simulink model "power_triphaseline"  (Simulink 6.0)
settings: Solver=ode15s  SolverMode=SingleTasking  StartTime=0.0  StopTime=0.1  RelTol=1e-3  AbsTol=1e-6
libraries: powerlib x17
settings Model: Creator=patrice  LastModifiedBy=batserve  ExtModeTrigMode=oneshot  ExtModeArmWhenConnect=off  ExtModeAutoUpdateStatusClock=off
settings DataIOCC: LimitDataPoints=off  SignalLoggingName=sigsOut
settings OptimizationCC: BlockReduction=off  BooleanDataType=off
settings DebuggingCC: CheckExecutionContextPreStartOutputMsg=on  CheckExecutionContextRuntimeOutputMsg=on  SolverPrmCheckMsg=none  IntegerOverflowMsg=none
settings HardwareCC: TargetUnknown=on
settings RTWCC: TemplateMakefile=grt_unix.tmf

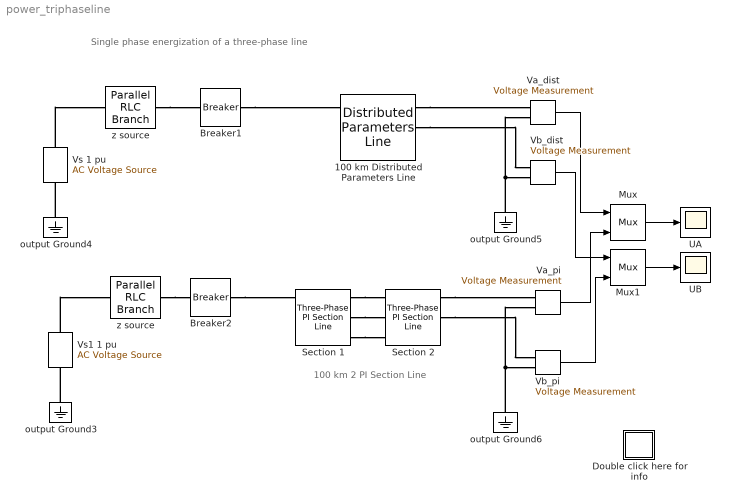
== system power_triphaseline ==
  note: 100 km
      | 2 PI Section Line
  note: Single phase energization of a three-phase line
  100 km Distributed Parameters Line : powerlib/Elements/Distributed Parameters Line  Phases=3  Frequency=60  Resistance=[0.01273 0.3864]  Inductance="[0.9337e-3  4.1264e-3]"  Capacitance=[12.74e-9 7.751e-9]  Length=100  x1=[0 0 0 0; 0.0001244 0 0 0; 0.0002488 0 0 0; 0.0003733 0 0 0; 0.0004977 0 0 0; 0.0006221 0 0 0]  x2=[0 0 0 0; 0.0001244 0 0 0; 0.0002488 0 0 0; 0.0003733 0 0 0; 0.0004977 0 0 0; 0.0006221 0 0 0]  x3=[0 0 0 0; 0.0001244 0 0 0; 0.0002488 0 0 0; 0.0003733 0 0 0; 0.0004977 0 0 0; 0.0006221 0 0 0]  x4=[0 0 0 0; 0.0001244 0 0 0; 0.0002488 0 0 0; 0.0003733 0 0 0; 0.0004977 0 0 0; 0.0006221 0 0 0]  x5=0  Measurements=None
      settings: AttributesFormatString=\n
  Breaker1 : powerlib/Elements/Breaker  BreakerResistance=0.01  InitialState=0  SnubberResistance=inf  SnubberCapacitance=0  SwitchingTimes="[ 0.25/60  4/60 ]"  External=off  Measurements=None
      settings: AttributesFormatString=\n
  Breaker2 : powerlib/Elements/Breaker  BreakerResistance=0.01  InitialState=0  SnubberResistance=inf  SnubberCapacitance=0  SwitchingTimes="[ .25/60  4/60 ]"  External=off  Measurements=None
      settings: AttributesFormatString=\n
  Double click here for info : Subsystem
      mask Display: disp('?')
  Mux : Mux  Inputs=2
  Mux1 : Mux  Inputs=2
  Section 1 : powerlib/Elements/Three-Phase PI Section Line  PhysicalDomain=powersysdomain  SubClassName=unknown  LeftPortType=p1  RightPortType=p1  LConnTagsString=a|b|c  RConnTagsString=A|B|C  Frequency=60  Resistances=[ 0.01273 0.3864]  Inductances="[ 0.9337e-3  4.1264e-3]"  Capacitances=[12.74e-9 7.751e-9]  Length=50
  Section 2 : powerlib/Elements/Three-Phase PI Section Line  PhysicalDomain=powersysdomain  SubClassName=unknown  LeftPortType=p1  RightPortType=p1  LConnTagsString=a|b|c  RConnTagsString=A|B|C  Frequency=60  Resistances=[ 0.01273 0.3864]  Inductances="[ 0.9337e-3  4.1264e-3]"  Capacitances=[12.74e-9 7.751e-9]  Length=50
  UA : Scope
      settings: TickLabels=on  TimeRange=0.1  YMin=-4  YMax=4  DataFormat=Array
  UB : Scope
      settings: TickLabels=on  TimeRange=0.1  YMin=-1  YMax=1  DataFormat=Array  MaxDataPoints=500000
  Va_dist : powerlib/Measurements/Voltage Measurement  Tag=PoWeRsYsTeMmEaSuReMeNt  PhasorSimulation=off  OutputType=Magnitude  PSBequivalent=0
  Va_pi : powerlib/Measurements/Voltage Measurement  Tag=PoWeRsYsTeMmEaSuReMeNt  PhasorSimulation=off  OutputType=Magnitude  PSBequivalent=0
  Vb_dist : powerlib/Measurements/Voltage Measurement  Tag=PoWeRsYsTeMmEaSuReMeNt  PhasorSimulation=off  OutputType=Magnitude  PSBequivalent=0
  Vb_pi : powerlib/Measurements/Voltage Measurement  Tag=PoWeRsYsTeMmEaSuReMeNt  PhasorSimulation=off  OutputType=Magnitude  PSBequivalent=0
  Vs 1 pu : powerlib/Electrical Sources/AC Voltage Source  Description=source block  Orientation=up  Amplitude=1  Phase=0  Frequency=60  SampleTime=0  Measurements=None
      settings: AttributesFormatString=\n
  Vs1 1 pu : powerlib/Electrical Sources/AC Voltage Source  Description=source block  Orientation=up  Amplitude=1  Phase=0  Frequency=60  SampleTime=0  Measurements=None
      settings: AttributesFormatString=\n
  output Ground{3..6} (4 alike) : powerlib/Elements/Ground  Orientation=down  PhysicalDomain=powersysdomain  SubClassName=unknown  LeftPortType=p1  RightPortType=p1  LConnTagsString=a
  z source : powerlib/Elements/Parallel RLC Branch  PhysicalDomain=powersysdomain  SubClassName=unknown  LeftPortType=p1  RightPortType=p1  LConnTagsString=a  RConnTagsString=__new0  Resistance=180  Inductance=47.8e-3  Capacitance=0  Measurements=None
  "z source " : powerlib/Elements/Parallel RLC Branch  PhysicalDomain=powersysdomain  SubClassName=unknown  LeftPortType=p1  RightPortType=p1  LConnTagsString=a  RConnTagsString=__new0  Resistance=180  Inductance=47.8e-3  Capacitance=0  Measurements=None
  wires:
  Mux1/1 -> UB/1
  Mux/1 -> UA/1
  Vb_dist/1 -> Mux1/1
  Va_dist/1 -> Mux/1
  Vb_pi/1 -> Mux1/2
  Va_pi/1 -> Mux/2
  connections:
  100 km Distributed Parameters Line/RConn1 -- Va_dist/LConn1
  100 km Distributed Parameters Line/RConn2 -- Vb_dist/LConn1
  output Ground5/LConn1 -- Vb_dist/LConn2 -- Va_dist/LConn2
  Breaker1/RConn1 -- 100 km Distributed Parameters Line/LConn1
  output Ground6/LConn1 -- Va_pi/LConn2 -- Vb_pi/LConn2
  Section 2/RConn2 -- Vb_pi/LConn1
  Section 2/RConn1 -- Va_pi/LConn1
  Section 1/RConn3 -- Section 2/LConn3
  Section 1/RConn2 -- Section 2/LConn2
  Section 1/RConn1 -- Section 2/LConn1
  Breaker2/RConn1 -- Section 1/LConn1
  "z source "/RConn1 -- Breaker2/LConn1
  z source/RConn1 -- Breaker1/LConn1
  output Ground4/LConn1 -- Vs 1 pu/LConn1
  Vs 1 pu/RConn1 -- z source/LConn1
  output Ground3/LConn1 -- Vs1 1 pu/LConn1
  Vs1 1 pu/RConn1 -- "z source "/LConn1

== system power_triphaseline/Double click here for info ==
  note: A 100 km, 3-phase line is energized on a 735 kV, 30,000 MVA  equivalent network.
      | The line is first energized on phase A at t = 1/4 cycle (maximum of source voltage) and then deenergized at t = 4 cycles.
      | Phase B and phase C are left open.
      | Switchings are performed simultaneously on two different line models:
      |
      | - Distributed Parameters Line
      | - Three-phase PI section Line consisting of two 50 km sections.
      |
      | Voltages obtained on phases A and B at the line receiving end with the two models are compared.
  note: This demonstration compares transients obtained with
      | a distributed parameter line model and a PI section line model
  note: Circuit Description
  note: Demonstration
  note: G. Sybille (Hydro-Quebec)
  note: Open the two scopes and start the simulation.
      | Compare the voltages obtained on phase A and phase B (induced voltage) with the two models.
      | Zoom on voltages rigth after energizing and notice the sharp edges obtained with the distributed parameter line (yellow trace).
      | These voltage steps which are due to travelling wave reflections at both ends  of the line are filtered by the PI model.
      | Notice also that phases A and B stay charged at peak voltage when the breakers are opened.
